simulink model "Assignment_11"  (R2019a)
settings: Solver=FixedStepDiscrete  StartTime=0.0  StopTime=100  FixedStep=1  RelTol=1e-3
settings Model: Creator=shara  LastModifiedBy=shara

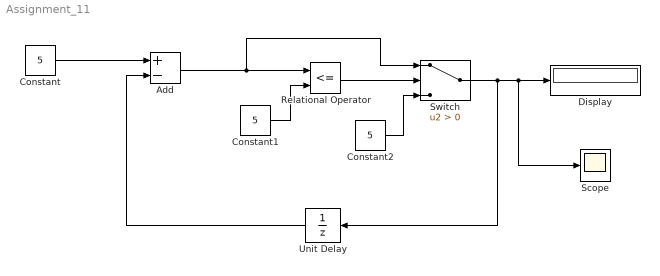
== system Assignment_11 ==
  Add : Sum  Inputs=+-
  Constant : Constant  Value=5
  Constant1 : Constant  Value=5
  Constant2 : Constant  Value=5
  Display : Display
  Relational Operator : RelationalOperator  Operator=<=  OutDataTypeStr=boolean  RndMeth=Simplest
  Scope : Scope
  Switch : Switch  Criteria=u2 > Threshold
  Unit Delay : UnitDelay  InitialCondition=1  SampleTime=-1  HasFrameUpgradeWarning=on
  wires:
  Constant/1 -> Add/1
  Add/1 -> Switch/1, Relational Operator/1
  Relational Operator/1 -> Switch/2
  Switch/1 -> Unit Delay/1, Scope/1, Display/1
  Unit Delay/1 -> Add/2
  Constant1/1 -> Relational Operator/2
  Constant2/1 -> Switch/3
